simulink model "pmsm_mpc_ekf"  (R2025b)
settings: Solver=ode23tb  StartTime=0.0  StopTime=simlength  FixedStep=tsample  MaxStep=ts
values from neighbouring files (symbols this model uses):
  ki_w = 1    [init.m]
  kp_w = 2    [init.m]
  simlength = 60    [init.m]
  tcontrol = 1/fPWM_INV/6    (= 2.08333333333e-05)    [init.m]
  ts = tcontrol    (= 2.08333333333e-05)    [init.m]
undefined symbols (not defined in the file or in its folder): A1_tilde, A2_tilde, A3_tilde, A4_tilde, Adrso, b, b_brake, Bd, C, Crso, ibez, Jm, Lalpha, Lbeta, Ldrso, omega_bez, omega_m_bez, omega_m_sim, psi_m, Qkalman, Rkalman, Rs, tau_bez, Vdc
libraries: fl_lib x19, nesl_utility x19, pmsm_alphabeta_lib x1, permanent_magnet_synchronous_machine x1
(part 2 of 2)

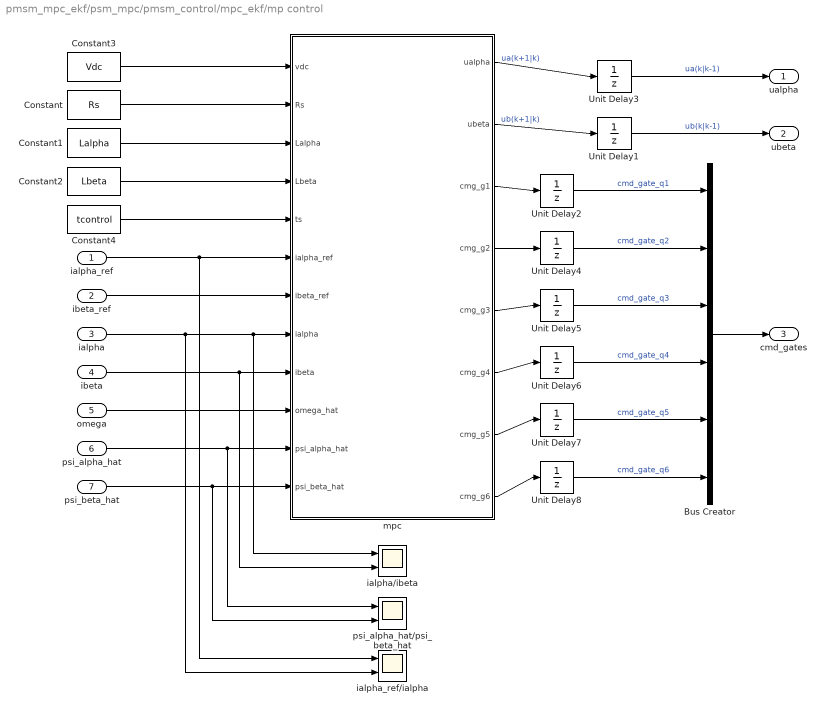
== system pmsm_mpc_ekf/psm_mpc/pmsm_control/mpc_ekf/mp control ==
  ialpha_ref : Inport
  ibeta_ref : Inport  Port=2
  ialpha : Inport  Port=3
  ibeta : Inport  Port=4
  omega : Inport  Port=5
  psi_alpha_hat : Inport  Port=6
  psi_beta_hat : Inport  Port=7
  Bus Creator : BusCreator  Inputs=6
  Constant : Constant  Value=Rs
  Constant1 : Constant  Value=Lalpha
  Constant2 : Constant  Value=Lbeta
  Constant3 : Constant  Value=Vdc
  Constant4 : Constant  Value=tcontrol
  Unit Delay{1..8} (8 alike) : UnitDelay  SampleTime=tcontrol  HasFrameUpgradeWarning=on
  ialpha/ibeta : Scope  NumInputPorts=2
      settings: SampleTime=ts  ActiveDisplayYMinimum=-1333.37712  ActiveDisplayYMaximum=1131.79846
  ialpha_ref/ialpha : Scope  NumInputPorts=2
      settings: SampleTime=ts  ActiveDisplayYMinimum=-1306.22726  ActiveDisplayYMaximum=1306.53939  DataLoggingVariableName=ScopeData2
  mpc : MATLAB Function  TreatAsAtomicUnit=on  SystemSampleTime=tcontrol
  psi_alpha_hat/psi_beta_hat : Scope  NumInputPorts=2
      settings: SampleTime=ts  ActiveDisplayYMinimum=-4.74729  ActiveDisplayYMaximum=4.18301
  ualpha : Outport
  ubeta : Outport  Port=2
  cmd_gates : Outport  Port=3
  wires:
  Constant2/1 -> mpc/4(Lbeta)
  psi_beta_hat/1 -> psi_alpha_hat/psi_beta_hat/2, mpc/12(psi_beta_hat)
  psi_alpha_hat/1 -> mpc/11(psi_alpha_hat), psi_alpha_hat/psi_beta_hat/1
  omega/1 -> mpc/10(omega_hat)
  mpc/2(ubeta) -> Unit Delay1/1  "ub(k+1|k)"
  Unit Delay1/1 -> ubeta/1  "ub(k|k-1)"
  ibeta/1 -> mpc/9(ibeta), ialpha/ibeta/2
  ialpha/1 -> ialpha_ref/ialpha/2, mpc/8(ialpha), ialpha/ibeta/1
  Constant4/1 -> mpc/5(ts)
  Constant3/1 -> mpc/1(vdc)
  Unit Delay3/1 -> ualpha/1  "ua(k|k-1)"
  mpc/1(ualpha) -> Unit Delay3/1  "ua(k+1|k)"
  Constant1/1 -> mpc/3(Lalpha)
  ibeta_ref/1 -> mpc/7(ibeta_ref)
  ialpha_ref/1 -> ialpha_ref/ialpha/1, mpc/6(ialpha_ref)
  Constant/1 -> mpc/2(Rs)
  mpc/8(cmg_g6) -> Unit Delay8/1
  mpc/7(cmg_g5) -> Unit Delay7/1
  mpc/6(cmg_g4) -> Unit Delay6/1
  mpc/5(cmg_g3) -> Unit Delay5/1
  mpc/4(cmg_g2) -> Unit Delay4/1
  mpc/3(cmg_g1) -> Unit Delay2/1
  Unit Delay2/1 -> Bus Creator/1  "cmd_gate_q1"
  Unit Delay4/1 -> Bus Creator/2  "cmd_gate_q2"
  Unit Delay5/1 -> Bus Creator/3  "cmd_gate_q3"
  Unit Delay6/1 -> Bus Creator/4  "cmd_gate_q4"
  Unit Delay7/1 -> Bus Creator/5  "cmd_gate_q5"
  Unit Delay8/1 -> Bus Creator/6  "cmd_gate_q6"
  Bus Creator/1 -> cmd_gates/1

== system pmsm_mpc_ekf/pmsm_ctrl/pmsm_control/mpc_ekf/extended kalman observer/A ==
  Gain1 : Gain  Gain=A2_tilde
  Gain{2,4,6,11} (4 alike) : Gain  Gain=tcontrol
  Gain3 : Gain  Gain=A3_tilde
  Gain5 : Gain  Gain=A4_tilde
  I1 : Constant  Value=eye(6)
  I2 : Constant  Value=A1_tilde
  Sum7 : Sum  Inputs=+++++
  out : Outport
  wires:
  Sum7/1 -> out/1
  I2/1 -> Gain11/1
  I1/1 -> Sum7/1
  Gain11/1 -> Sum7/2
  Gain1/1 -> Gain2/1
  Gain2/1 -> Sum7/3
  Gain3/1 -> Gain4/1
  Gain4/1 -> Sum7/4
  Gain5/1 -> Gain6/1
  Gain6/1 -> Sum7/5
  [omega_hat_kalman] -> Gain1/1
  [psi_alpha_hat] -> Gain3/1
  [psi_beta_hat] -> Gain5/1

== system pmsm_mpc_ekf/pmsm_ctrl/pmsm_control/mpc_ekf/extended kalman observer/A  ==
  Gain1 : Gain  Gain=A2_tilde
  Gain{2,4,6,11} (4 alike) : Gain  Gain=tcontrol
  Gain3 : Gain  Gain=A3_tilde
  Gain5 : Gain  Gain=A4_tilde
  I1 : Constant  Value=eye(6)
  I2 : Constant  Value=A1_tilde
  Sum7 : Sum  Inputs=+++++
  out : Outport
  wires:
  [psi_beta_hat] -> Gain5/1
  [psi_alpha_hat] -> Gain3/1
  [omega_hat_kalman] -> Gain1/1
  Gain6/1 -> Sum7/5
  Gain5/1 -> Gain6/1
  Gain4/1 -> Sum7/4
  Gain3/1 -> Gain4/1
  Gain2/1 -> Sum7/3
  Gain1/1 -> Gain2/1
  Gain11/1 -> Sum7/2
  I1/1 -> Sum7/1
  I2/1 -> Gain11/1
  Sum7/1 -> out/1

== system pmsm_mpc_ekf/psm_mpc/pmsm_control/mpc_ekf/extended kalman observer/A ==
  Gain1 : Gain  Gain=A2_tilde
  Gain{2,4,6,11} (4 alike) : Gain  Gain=tcontrol
  Gain3 : Gain  Gain=A3_tilde
  Gain5 : Gain  Gain=A4_tilde
  I1 : Constant  Value=eye(6)
  I2 : Constant  Value=A1_tilde
  Sum7 : Sum  Inputs=+++++
  out : Outport
  wires:
  [psi_beta_hat] -> Gain5/1
  [psi_alpha_hat] -> Gain3/1
  [omega_hat_kalman] -> Gain1/1
  Gain6/1 -> Sum7/5
  Gain5/1 -> Gain6/1
  Gain4/1 -> Sum7/4
  Gain3/1 -> Gain4/1
  Gain2/1 -> Sum7/3
  Gain1/1 -> Gain2/1
  Gain11/1 -> Sum7/2
  I1/1 -> Sum7/1
  I2/1 -> Gain11/1
  Sum7/1 -> out/1

== system pmsm_mpc_ekf/psm_mpc/pmsm_control/mpc_ekf/extended kalman observer/A  ==
  Gain1 : Gain  Gain=A2_tilde
  Gain{2,4,6,11} (4 alike) : Gain  Gain=tcontrol
  Gain3 : Gain  Gain=A3_tilde
  Gain5 : Gain  Gain=A4_tilde
  I1 : Constant  Value=eye(6)
  I2 : Constant  Value=A1_tilde
  Sum7 : Sum  Inputs=+++++
  out : Outport
  wires:
  Sum7/1 -> out/1
  I2/1 -> Gain11/1
  I1/1 -> Sum7/1
  Gain11/1 -> Sum7/2
  Gain1/1 -> Gain2/1
  Gain2/1 -> Sum7/3
  Gain3/1 -> Gain4/1
  Gain4/1 -> Sum7/4
  Gain5/1 -> Gain6/1
  Gain6/1 -> Sum7/5
  [omega_hat_kalman] -> Gain1/1
  [psi_alpha_hat] -> Gain3/1
  [psi_beta_hat] -> Gain5/1

== matlab function pmsm_mpc_ekf/pmsm_ctrl/pmsm_control/double_integrator_observer/bounder1 ==
  data: u input; y output
function y = bounder(u)
    
    u = -pi + mod(u+3*pi,2*pi);
    
    y = u;
end

== matlab function pmsm_mpc_ekf/psm_mpc/pmsm_control/double_integrator_observer/bounder1 ==
  data: u input; y output
function y = bounder(u)
    
    u = -pi + mod(u+3*pi,2*pi);
    
    y = u;
end

== matlab function pmsm_mpc_ekf/pmsm_ctrl/pmsm_control/double_integrator_observer/bounder2 ==
  data: u input; y output
function y = bounder(u)
    
    u = -pi + mod(u+3*pi,2*pi);
    
    y = u;
end

== matlab function pmsm_mpc_ekf/pmsm_ctrl/pmsm_control/mpc_ekf/mp control/mpc ==
  data: vdc input; Rs input; Lalpha input; Lbeta input; ts input; ialpha_ref input; ibeta_ref input; ialpha input; ualpha output; ibeta input; omega_hat input; psi_alpha_hat input; psi_beta_hat input; ubeta output
function [ualpha, ubeta]    = mpc(vdc, Rs, Lalpha, Lbeta, ts, ialpha_ref,...
    ibeta_ref, ialpha, ibeta, omega_hat, psi_alpha_hat, psi_beta_hat)

    persistent ualpha_z ubeta_z

    ualpha_1 = 2/3*vdc;
    ubeta_1 = 0;

    ualpha_2 = 2/3*1/2*vdc;
    ubeta_2 = 2/3*sqrt(3)/2*vdc;

    ualpha_3 = -2/3*1/2*vdc;
    ubeta_3 = 2/3*sqrt(3)/2*vdc;

    ualpha_4 = -2/3*vdc;
    ubeta_4 = 0;

    ualpha_5 = -2/3*1/2*vdc;
    ubeta_5 = -2/3*sqrt(3)/2*vdc;

    ualpha_6 = 2/3*1/2*vdc;
    ubeta_6 = -2/3*sqrt(3)/2*vdc;

    ualpha_0 = 0;
    ubeta_0 = 0;

    if isempty(ualpha_z)
        ualpha_z = 0;
        ubeta_z = 0;
    end

    ia_p0 = (1-Rs/Lalpha*ts)*ialpha + omega_hat/Lalpha*psi_beta_hat*ts + ualpha_0*ts/Lalpha;
    ib_p0 = (1-Rs/Lbeta*ts)*ibeta - omega_hat/Lbeta*psi_alpha_hat*ts + ubeta_0*ts/Lbeta;
    
    ia_p1 = (1-Rs/Lalpha*ts)*ialpha + omega_hat/Lalpha*psi_beta_hat*ts + ualpha_1*ts/Lalpha;
    ib_p1 = (1-Rs/Lbeta*ts)*ibeta - omega_hat/Lbeta*psi_alpha_hat*ts + ubeta_1*ts/Lbeta;

    ia_p2 = (1-Rs/Lalpha*ts)*ialpha + omega_hat/Lalpha*psi_beta_hat*ts + ualpha_2*ts/Lalpha;
    ib_p2 = (1-Rs/Lbeta*ts)*ibeta - omega_hat/Lbeta*psi_alpha_hat*ts + ubeta_2*ts/Lbeta;

    ia_p3 = (1-Rs/Lalpha*ts)*ialpha + omega_hat/Lalpha*psi_beta_hat*ts + ualpha_3*ts/Lalpha;
    ib_p3 = (1-Rs/Lbeta*ts)*ibeta - omega_hat/Lbeta*psi_alpha_hat*ts + ubeta_3*ts/Lbeta;

    ia_p4 = (1-Rs/Lalpha*ts)*ialpha + omega_hat/Lalpha*psi_beta_hat*ts + ualpha_4*ts/Lalpha;
    ib_p4 = (1-Rs/Lbeta*ts)*ibeta - omega_hat/Lbeta*psi_alpha_hat*ts + ubeta_4*ts/Lbeta;

    ia_p5 = (1-Rs/Lalpha*ts)*ialpha + omega_hat/Lalpha*psi_beta_hat*ts + ualpha_5*ts/Lalpha;
    ib_p5 = (1-Rs/Lbeta*ts)*ibeta - omega_hat/Lbeta*psi_alpha_hat*ts + ubeta_5*ts/Lbeta;

    ia_p6 = (1-Rs/Lalpha*ts)*ialpha + omega_hat/Lalpha*psi_beta_hat*ts + ualpha_6*ts/Lalpha;
    ib_p6 = (1-Rs/Lbeta*ts)*ibeta - omega_hat/Lbeta*psi_alpha_hat*ts + ubeta_6*ts/Lbeta;
  
    J0 = (ialpha_ref - ia_p0)^2 + (ibeta_ref - ib_p0)^2;
    J1 = (ialpha_ref - ia_p1)^2 + (ibeta_ref - ib_p1)^2;
    J2 = (ialpha_ref - ia_p2)^2 + (ibeta_ref - ib_p2)^2;
    J3 = (ialpha_ref - ia_p3)^2 + (ibeta_ref - ib_p3)^2;
    J4 = (ialpha_ref - ia_p4)^2 + (ibeta_ref - ib_p4)^2;
    J5 = (ialpha_ref - ia_p5)^2 + (ibeta_ref - ib_p5)^2;
    J6 = (ialpha_ref - ia_p6)^2 + (ibeta_ref - ib_p6)^2;
    
    if (ualpha_z == ualpha_0) && (ubeta_z == ubeta_0)
        [m,i] = min([J0, J1, J2, J3, J4, J5, J6]);
        if i == 1
            ualpha = ualpha_0;
            ubeta = ubeta_0;
        elseif i == 2
            ualpha = ualpha_1;
            ubeta = ubeta_1;
        elseif i == 3
            ualpha = ualpha_2;
            ubeta = ubeta_2;
        elseif i == 4
            ualpha = ualpha_3;
            ubeta = ubeta_3;
        elseif i == 5
            ualpha = ualpha_4;
            ubeta = ubeta_4;
        elseif i == 6
            ualpha = ualpha_5;
            ubeta = ubeta_5;
        else
            ualpha = ualpha_6;
            ubeta = ubeta_6;
        end
    elseif (ualpha_z == ualpha_1) && (ubeta_z == ubeta_1)
        [m,i] = min([J0, J1, J2, J6]);
        if i == 1
            ualpha = ualpha_0;
            ubeta = ubeta_0;
        elseif i == 2
            ualpha = ualpha_1;
            ubeta = ubeta_1;
        elseif i == 3
            ualpha = ualpha_2;
            ubeta = ubeta_2;
        else
            ualpha = ualpha_6;
            ubeta = ubeta_6;
        end
    elseif (ualpha_z == ualpha_2) && (ubeta_z == ubeta_2) % vector u2
        [m,i] = min([J0, J1, J2, J3]);
        if i == 1
            ualpha = ualpha_0;
            ubeta = ubeta_0;
        elseif i == 2
            ualpha = ualpha_1;
            ubeta = ubeta_1;
        elseif i == 3
            ualpha = ualpha_2;
            ubeta = ubeta_2;
        else
            ualpha = ualpha_3;
            ubeta = ubeta_3;
        end
    elseif (ualpha_z == ualpha_3) && (ubeta_z == ubeta_3)
        [m,i] = min([J0, J2, J3, J4]);
        if i == 1
            ualpha = ualpha_0;
            ubeta = ubeta_0;
        elseif i == 2
            ualpha = ualpha_2;
            ubeta = ubeta_2;
        elseif i == 3
            ualpha = ualpha_3;
            ubeta = ubeta_3;
        else
            ualpha = ualpha_4;
            ubeta = ubeta_4;
        end
    elseif (ualpha_z == ualpha_4) && (ubeta_z == ubeta_4)
        [m,i] = min([J0, J3, J4, J5]);
        if i == 1
            ualpha = ualpha_0;
            ubeta = ubeta_0;
        elseif i == 2
            ualpha = ualpha_3;
            ubeta = ubeta_3;
        elseif i == 3
            ualpha = ualpha_4;
            ubeta = ubeta_4;
        else
            ualpha = ualpha_5;
            ubeta = ubeta_5;
        end
    elseif (ualpha_z == ualpha_5) && (ubeta_z == ubeta_5) % u5
        [m,i] = min([J0, J4, J5, J6]);
        if i == 1
            ualpha = ualpha_0;
            ubeta = ubeta_0;
        elseif i == 2
            ualpha = ualpha_4;
            ubeta = ubeta_4;
        elseif i == 3
            ualpha = ualpha_5;
            ubeta = ubeta_5;
        else
            ualpha = ualpha_6;
            ubeta = ubeta_6;
        end
    else
        [m,i] = min([J0, J5, J6, J1]);
        if i == 1
            ualpha = ualpha_0;
            ubeta = ubeta_0;
        elseif i == 2
            ualpha = ualpha_5;
            ubeta = ubeta_5;
        elseif i == 3
            ualpha = ualpha_6;
            ubeta = ubeta_6;
        else
            ualpha = ualpha_1;
            ubeta = ubeta_1;
        end
    end
    ualpha_z = ualpha;
    ubeta_z = ubeta;
end

== matlab function pmsm_mpc_ekf/psm_mpc/pmsm_control/double_integrator_observer/bounder2 ==
  data: u input; y output
function y = bounder(u)
    
    u = -pi + mod(u+3*pi,2*pi);
    
    y = u;
end

== matlab function pmsm_mpc_ekf/psm_mpc/pmsm_control/mpc_ekf/mp control/mpc ==
  data: vdc input; Rs input; Lalpha input; Lbeta input; ts input; ialpha_ref input; ibeta_ref input; ialpha input; ualpha output; ibeta input; omega_hat input; psi_alpha_hat input; psi_beta_hat input; ubeta output; cmg_g1 output; cmg_g2 output; cmg_g3 output; cmg_g4 output; cmg_g5 output; cmg_g6 output
function [ualpha, ubeta, cmg_g1, cmg_g2, cmg_g3, cmg_g4, cmg_g5, cmg_g6]    = mpc(vdc, Rs, Lalpha, Lbeta, ts, ialpha_ref,...
    ibeta_ref, ialpha, ibeta, omega_hat, psi_alpha_hat, psi_beta_hat)

    persistent ualpha_z ubeta_z

    on = vdc;
    off = 0;

    ualpha_1 = 2/3*vdc;
    ubeta_1 = 0;

    ualpha_2 = 2/3*1/2*vdc;
    ubeta_2 = 2/3*sqrt(3)/2*vdc;

    ualpha_3 = -2/3*1/2*vdc;
    ubeta_3 = 2/3*sqrt(3)/2*vdc;

    ualpha_4 = -2/3*vdc;
    ubeta_4 = 0;

    ualpha_5 = -2/3*1/2*vdc;
    ubeta_5 = -2/3*sqrt(3)/2*vdc;

    ualpha_6 = 2/3*1/2*vdc;
    ubeta_6 = -2/3*sqrt(3)/2*vdc;

    ualpha_0 = 0;
    ubeta_0 = 0;

    if isempty(ualpha_z)
        ualpha_z = 0;
        ubeta_z = 0;
    end

    ia_p0 = (1-Rs/Lalpha*ts)*ialpha + omega_hat/Lalpha*psi_beta_hat*ts + ualpha_0*ts/Lalpha;
    ib_p0 = (1-Rs/Lbeta*ts)*ibeta - omega_hat/Lbeta*psi_alpha_hat*ts + ubeta_0*ts/Lbeta;
    
    ia_p1 = (1-Rs/Lalpha*ts)*ialpha + omega_hat/Lalpha*psi_beta_hat*ts + ualpha_1*ts/Lalpha;
    ib_p1 = (1-Rs/Lbeta*ts)*ibeta - omega_hat/Lbeta*psi_alpha_hat*ts + ubeta_1*ts/Lbeta;

    ia_p2 = (1-Rs/Lalpha*ts)*ialpha + omega_hat/Lalpha*psi_beta_hat*ts + ualpha_2*ts/Lalpha;
    ib_p2 = (1-Rs/Lbeta*ts)*ibeta - omega_hat/Lbeta*psi_alpha_hat*ts + ubeta_2*ts/Lbeta;

    ia_p3 = (1-Rs/Lalpha*ts)*ialpha + omega_hat/Lalpha*psi_beta_hat*ts + ualpha_3*ts/Lalpha;
    ib_p3 = (1-Rs/Lbeta*ts)*ibeta - omega_hat/Lbeta*psi_alpha_hat*ts + ubeta_3*ts/Lbeta;

    ia_p4 = (1-Rs/Lalpha*ts)*ialpha + omega_hat/Lalpha*psi_beta_hat*ts + ualpha_4*ts/Lalpha;
    ib_p4 = (1-Rs/Lbeta*ts)*ibeta - omega_hat/Lbeta*psi_alpha_hat*ts + ubeta_4*ts/Lbeta;

    ia_p5 = (1-Rs/Lalpha*ts)*ialpha + omega_hat/Lalpha*psi_beta_hat*ts + ualpha_5*ts/Lalpha;
    ib_p5 = (1-Rs/Lbeta*ts)*ibeta - omega_hat/Lbeta*psi_alpha_hat*ts + ubeta_5*ts/Lbeta;

    ia_p6 = (1-Rs/Lalpha*ts)*ialpha + omega_hat/Lalpha*psi_beta_hat*ts + ualpha_6*ts/Lalpha;
    ib_p6 = (1-Rs/Lbeta*ts)*ibeta - omega_hat/Lbeta*psi_alpha_hat*ts + ubeta_6*ts/Lbeta;
  
    J0 = (ialpha_ref - ia_p0)^2 + (ibeta_ref - ib_p0)^2;
    J1 = (ialpha_ref - ia_p1)^2 + (ibeta_ref - ib_p1)^2;
    J2 = (ialpha_ref - ia_p2)^2 + (ibeta_ref - ib_p2)^2;
    J3 = (ialpha_ref - ia_p3)^2 + (ibeta_ref - ib_p3)^2;
    J4 = (ialpha_ref - ia_p4)^2 + (ibeta_ref - ib_p4)^2;
    J5 = (ialpha_ref - ia_p5)^2 + (ibeta_ref - ib_p5)^2;
    J6 = (ialpha_ref - ia_p6)^2 + (ibeta_ref - ib_p6)^2;
    
    if (ualpha_z == ualpha_0) && (ubeta_z == ubeta_0)
        [m,i] = min([J0, J1, J2, J3, J4, J5, J6]);
        if i == 1
            ualpha = ualpha_0;
            ubeta = ubeta_0;
        elseif i == 2
            ualpha = ualpha_1;
            ubeta = ubeta_1;
        elseif i == 3
            ualpha = ualpha_2;
            ubeta = ubeta_2;
        elseif i == 4
            ualpha = ualpha_3;
            ubeta = ubeta_3;
        elseif i == 5
            ualpha = ualpha_4;
            ubeta = ubeta_4;
        elseif i == 6
            ualpha = ualpha_5;
            ubeta = ubeta_5;
        else
            ualpha = ualpha_6;
            ubeta = ubeta_6;
        end
    elseif (ualpha_z == ualpha_1) && (ubeta_z == ubeta_1)
        [m,i] = min([J0, J1, J2, J6]);
        if i == 1
            ualpha = ualpha_0;
            ubeta = ubeta_0;
        elseif i == 2
            ualpha = ualpha_1;
            ubeta = ubeta_1;
        elseif i == 3
            ualpha = ualpha_2;
            ubeta = ubeta_2;
        else
            ualpha = ualpha_6;
            ubeta = ubeta_6;
        end
    elseif (ualpha_z == ualpha_2) && (ubeta_z == ubeta_2) % vector u2
        [m,i] = min([J0, J1, J2, J3]);
        if i == 1
            ualpha = ualpha_0;
            ubeta = ubeta_0;
        elseif i == 2
            ualpha = ualpha_1;
            ubeta = ubeta_1;
        elseif i == 3
            ualpha = ualpha_2;
            ubeta = ubeta_2;
        else
            ualpha = ualpha_3;
            ubeta = ubeta_3;
        end
    elseif (ualpha_z == ualpha_3) && (ubeta_z == ubeta_3)
        [m,i] = min([J0, J2, J3, J4]);
        if i == 1
            ualpha = ualpha_0;
            ubeta = ubeta_0;
        elseif i == 2
            ualpha = ualpha_2;
            ubeta = ubeta_2;
        elseif i == 3
            ualpha = ualpha_3;
            ubeta = ubeta_3;
        else
            ualpha = ualpha_4;
            ubeta = ubeta_4;
        end
    elseif (ualpha_z == ualpha_4) && (ubeta_z == ubeta_4)
        [m,i] = min([J0, J3, J4, J5]);
        if i == 1
            ualpha = ualpha_0;
            ubeta = ubeta_0;
        elseif i == 2
            ualpha = ualpha_3;
            ubeta = ubeta_3;
        elseif i == 3
            ualpha = ualpha_4;
            ubeta = ubeta_4;
        else
            ualpha = ualpha_5;
            ubeta = ubeta_5;
        end
    elseif (ualpha_z == ualpha_5) && (ubeta_z == ubeta_5) % u5
        [m,i] = min([J0, J4, J5, J6]);
        if i == 1
            ualpha = ualpha_0;
            ubeta = ubeta_0;
        elseif i == 2
            ualpha = ualpha_4;
            ubeta = ubeta_4;
        elseif i == 3
            ualpha = ualpha_5;
            ubeta = ubeta_5;
        else
            ualpha = ualpha_6;
            ubeta = ubeta_6;
        end
    else
        [m,i] = min([J0, J5, J6, J1]);
        if i == 1
            ualpha = ualpha_0;
            ubeta = ubeta_0;
        elseif i == 2
            ualpha = ualpha_5;
            ubeta = ubeta_5;
        elseif i == 3
            ualpha = ualpha_6;
            ubeta = ubeta_6;
        else
            ualpha = ualpha_1;
            ubeta = ubeta_1;
        end
    end
    ualpha_z = ualpha;
    ubeta_z = ubeta;

    if (ualpha == ualpha_0 && ubeta == ubeta_0)
        cmg_g1 = on;
        cmg_g2 = off;
        cmg_g3 = on;
        cmg_g4 = off;
        cmg_g5 = on;
        cmg_g6 = off;
    elseif (ualpha == ualpha_1 && ubeta == ubeta_1)
        cmg_g1 = on;
        cmg_g2 = off;
        cmg_g3 = off;
        cmg_g4 = on;
        cmg_g5 = off;
        cmg_g6 = on;
    elseif (ualpha == ualpha_2 && ubeta == ubeta_2)
        cmg_g1 = on;
        cmg_g2 = off;
        cmg_g3 = on;
        cmg_g4 = off;
        cmg_g5 = off;
        cmg_g6 = on;
    elseif (ualpha == ualpha_3 && ubeta == ubeta_3)
        cmg_g1 = off;
        cmg_g2 = on;
        cmg_g3 = on;
        cmg_g4 = off;
        cmg_g5 = off;
        cmg_g6 = on;
    elseif (ualpha == ualpha_4 && ubeta == ubeta_4)
        cmg_g1 = off;
        cmg_g2 = on;
        cmg_g3 = on;
        cmg_g4 = off;
        cmg_g5 = on;
        cmg_g6 = off;
    elseif (ualpha == ualpha_5 && ubeta == ubeta_5)
        cmg_g1 = off;
        cmg_g2 = on;
        cmg_g3 = off;
        cmg_g4 = on;
        cmg_g5 = on;
        cmg_g6 = off;
    else
        cmg_g1 = on;
        cmg_g2 = off;
        cmg_g3 = off;
        cmg_g4 = on;
        cmg_g5 = on;
        cmg_g6 = off;
    end  
end
